simulink model "simReadEDF"  (R2018a)
settings: Solver=VariableStepAuto  StartTime=0.0  StopTime=10.0  RelTol=1e-3
settings Model: EnablePacing=on  Creator=User  LastModifiedBy=User

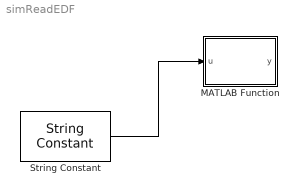
== system simReadEDF ==
  MATLAB Function : MATLAB Function  TreatAsAtomicUnit=on
  String Constant : StringConstant  String="\"C:\\Users\\User\\Documents\\GitHub\\MEng-Project\\Dataset (physionet.org-pn4-eegmmidb)\\RawData\\S001R01.edf\""
  wires:
  String Constant/1 -> MATLAB Function/1(u)

== matlab function simReadEDF/MATLAB Function ==
  data: u input; y output
function y = fcn(u)
EDFFilePath = 'C:\Users\User\Documents\GitHub\MEng-Project\Dataset (physionet.org-pn4-eegmmidb)\RawData\S001R01.edf'
EDFData = ReadEDF(EDFFilePath);
y = u;
